simulink model "Elevator"  (R2014a)
settings: Solver=ode45  StartTime=0.0  StopTime=10.0  RelTol=1e-3
libraries: simulink x2
settings Model: Creator=Rishabh  LastModifiedBy=Rishabh
settings DataIOCC: InspectSignalLogs=on

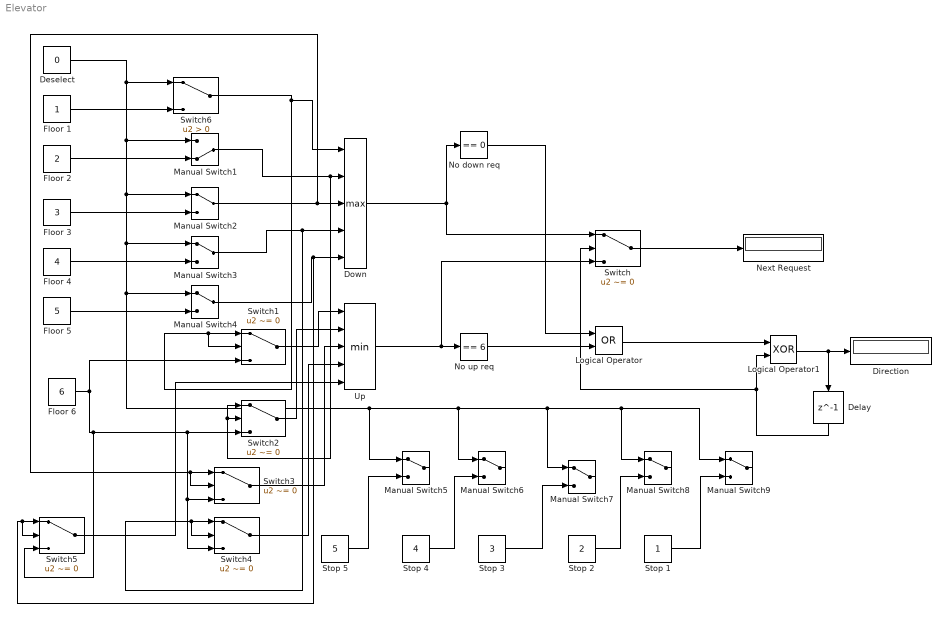
== system Elevator ==
  Delay : Delay  DelayLength=1  InitialCondition=0  SampleTime=1
  Deselect : Constant  Value=0
  Direction : Display
  Down : MinMax  Function=max  Inputs=5
  Floor 1 : Constant
  Floor 2 : Constant  Value=2
  Floor 3 : Constant  Value=3
  Floor 4 : Constant  Value=4
  Floor 5 : Constant  Value=5
  Floor 6 : Constant  Value=6
  Logical Operator : Logic  Operator=OR  AllPortsSameDT=off  OutDataTypeStr=boolean
  Logical Operator1 : Logic  Operator=XOR  AllPortsSameDT=off  OutDataTypeStr=boolean
  Manual Switch1 : ManualSwitch  CurrentSetting=0
  Manual Switch{2..9} (8 alike) : ManualSwitch
  Next Request : Display
  No down req : simulink/Logic and Bit Operations/Compare To Constant  relop===  const=0  OutDataTypeStr=boolean
  No up req : simulink/Logic and Bit Operations/Compare To Constant  relop===  const=6  OutDataTypeStr=boolean
  Stop 1 : Constant
  Stop 2 : Constant  Value=2
  Stop 3 : Constant  Value=3
  Stop 4 : Constant  Value=4
  Stop 5 : Constant  Value=5
  Switch : Switch  Criteria=u2 ~= 0
  Switch{1..5} (5 alike) : Switch  Criteria=u2 ~= 0  Threshold=5
  Switch6 : Switch  Criteria=u2 > Threshold
  Up : MinMax  Inputs=5
  wires:
  Floor 1/1 -> Switch6/3
  Floor 2/1 -> Manual Switch1/2
  Floor 3/1 -> Manual Switch2/2
  Floor 4/1 -> Manual Switch3/2
  Floor 5/1 -> Manual Switch4/2
  Deselect/1 -> Switch6/1, Manual Switch3/1, Manual Switch5/1, Manual Switch6/1, Manual Switch7/1, Manual Switch8/1, Manual Switch9/1, Manual Switch4/1, Manual Switch2/1, Manual Switch1/1
  Switch6/1 -> Switch1/2, Switch1/1, Down/1
  Manual Switch2/1 -> Switch3/2, Switch3/1, Down/3
  Manual Switch3/1 -> Down/4, Switch4/2, Switch4/1
  Manual Switch4/1 -> Switch5/2, Switch5/1, Down/5
  Stop 5/1 -> Manual Switch5/2
  Stop 4/1 -> Manual Switch6/2
  Stop 3/1 -> Manual Switch7/2
  Stop 2/1 -> Manual Switch8/2
  Stop 1/1 -> Manual Switch9/2
  Down/1 -> Switch/1, No down req/1
  Up/1 -> Switch/3, No up req/1
  Switch/1 -> Next Request/1
  Manual Switch1/1 -> Switch2/1, Switch2/2, Down/2
  Switch1/1 -> Up/1
  Floor 6/1 -> Switch5/3, Switch4/3, Switch3/3, Switch2/3, Switch1/3
  Switch2/1 -> Up/2
  Switch3/1 -> Up/3
  Switch4/1 -> Up/4
  Switch5/1 -> Up/5
  No up req/1 -> Logical Operator/2
  No down req/1 -> Logical Operator/1
  Logical Operator1/1 -> Delay/1, Direction/1
  Logical Operator/1 -> Logical Operator1/1
  Delay/1 -> Logical Operator1/2, Switch/2
